simulink model "lab5machine"  (R2019b)
settings: Solver=FixedStepAuto  StartTime=0  StopTime=0.2  FixedStep=0.0001  RelTol=1e-3
values from neighbouring files (symbols this model uses):
  B = 0.01    [lab5.m]
  f = 50    [lab5.m]
  J = 0.1    [lab5.m]
  Lr = (2.2+(N/3.5e3))/1000    (= 0.00465628571429)    [lab5.m]
  Ls = (2.5+(N/4e3))/1000    (= 0.00464925)    [lab5.m]
  P = (8e3-(N/2))    (= 3701.5)    [lab5.m]
  phase = 0    [lab5.m]
  Pp = 2    [lab5.m]
  Rr = (0.3+(N/20e3))    (= 0.72985)    [lab5.m]
  Rs = (0.4+(N/15e3))    (= 0.973133333333)    [lab5.m]
  V = 400    [lab5.m]
libraries: powerlib x9
settings Model: Creator=robom  LastModifiedBy=robom
settings DataIOCC: SaveOutput=off  ReturnWorkspaceOutputs=off

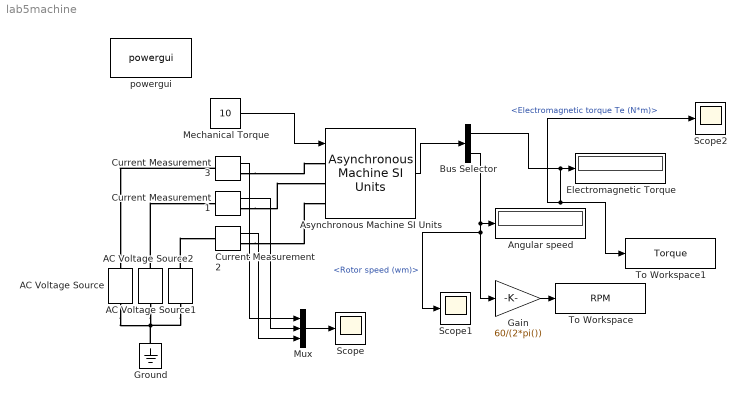
== system lab5machine ==
  AC Voltage Source : powerlib/Electrical Sources/AC Voltage Source  Amplitude=(V*sqrt(2))/sqrt(3)  Phase=phase  Frequency=f  SampleTime=0  Measurements=None  BusType=swing  Pref=10e3  Qref=0  Qmin=-inf  Qmax=+inf
      settings: SourceProductName=Simscape Electrical
  AC Voltage Source1 : powerlib/Electrical Sources/AC Voltage Source  Amplitude=(V*sqrt(2))/sqrt(3)  Phase=phase-120  Frequency=f  SampleTime=0  Measurements=None  BusType=swing  Pref=10e3  Qref=0  Qmin=-inf  Qmax=+inf
      settings: SourceProductName=Simscape Electrical
  AC Voltage Source2 : powerlib/Electrical Sources/AC Voltage Source  Amplitude=(V*sqrt(2))/sqrt(3)  Phase=phase+120  Frequency=f  SampleTime=0  Measurements=None  BusType=swing  Pref=10e3  Qref=0  Qmin=-inf  Qmax=+inf
      settings: SourceProductName=Simscape Electrical
  Angular speed : Display
  Asynchronous Machine SI Units : powerlib/Machines/Asynchronous Machine SI Units  RotorType=Squirrel-cage  PresetModel=No  MechanicalLoad=Torque Tm  ShowDetailedParameters=on  ReferenceFrame=Synchronous  Units=SI  MeasurementBus=off  NominalParameters=[P V f]  Stator=[Rs Ls]  Rotor=[Rr Lr]  Cage1=[0.4155 0.002066]  Cage2=[0.4168 0.0003495]  Lm=Lm  Mechanical=[J B Pp]  PolePairs=2  InitialConditions=[0 0 0 0 0 0 0 0]  SimulateSaturation=off  Saturation=[14.03593122, 27.81365428, 53.79336849, 72.68890987, 97.98006896, 148.6815601, 215.7428561, 302.9841135, 428.7778367 ; 230, 322, 414, 460, 506, 552, 598, 644, 690]  LoadFlowParameters=1492000  TsPowergui=0  TsBlock=-1  IterativeModel=Trapezoidal non iterative  IterativeDiscreteModel=Trapezoidal non iterative  Pmec=1.492e+006
      settings: SourceProductName=Simscape Electrical
  Bus Selector : BusSelector  OutputSignals=Mechanical.Electromagnetic torque Te (N*m),Mechanical.Rotor speed (wm)
  Current Measurement1 : powerlib/Measurements/Current Measurement  PhasorSimulation=off  OutputType=Complex  PSBequivalent=0
      settings: SourceProductName=Simscape Electrical
  Current Measurement2 : powerlib/Measurements/Current Measurement  PhasorSimulation=off  OutputType=Complex  PSBequivalent=0
      settings: SourceProductName=Simscape Electrical
  Current Measurement3 : powerlib/Measurements/Current Measurement  PhasorSimulation=off  OutputType=Complex  PSBequivalent=0
      settings: SourceProductName=Simscape Electrical
  Electromagnetic Torque : Display
  Gain : Gain  Gain=60/(2*pi())
  Ground : powerlib/Elements/Ground  LConnTagsString=a
      settings: SourceProductName=Simscape Electrical
  Mechanical Torque : Constant  Value=10
  Mux : Mux  Inputs=3
  Scope : Scope
  Scope1 : Scope
  Scope2 : Scope
  To Workspace : ToWorkspace  VariableName=RPM  SampleTime=-1
      settings: Save2DSignal=2-D array (concatenate along first dimension)
  To Workspace1 : ToWorkspace  VariableName=Torque  SampleTime=-1
      settings: Save2DSignal=2-D array (concatenate along first dimension)
  powergui : powerlib/powergui  Priority=1  SimulationMode=Continuous  SampleTime=50e-6  frequency=60  Iterations=50  frequencyindice=50  Pbase=100e6  ErrMax=1e-4  UnitsV=kV  UnitsW=MW  buscounter=0  FunctionMessages=off  echomessages=off  EnableUseOfTLC=off  CurrentSourceSwitches=off  DisableSnubberDevices=off  DisableRonSwitches=off  DisableVfSwitches=off  DisplayEquations=off  AutomaticDiscreteSolvers=off  SolverType=Tustin/Backward Euler (TBE)  Interpol=off  ExternalGateDelay=off  methode=off  Ts=100  x0status=blocks  SPID=on  SwTol=0  HookPort=off  NonlinearTolerance=1e-4  nMaxIteration=100  ContinueOnMaxIteration=off  RestoreLinks=warning  ResistiveCurrentMeasurement=off  Frange=[0:2:500]  Ylog=off  Xlog=on  ShowGrid=off  save=off  variable=ZData  structure=0  ZoomFFT=off  StartTime=0.0  cycles=1  DisplayStyle=1  fundamental=60  FreqAxis=off  MaxFrequency=1000  frequencyindicesteady=1  RmsSteady=1  display=off
      settings: SourceProductName=Simscape Electrical
  wires:
  Mechanical Torque/1 -> Asynchronous Machine SI Units/1
  Current Measurement2/1 -> Mux/3
  Current Measurement1/1 -> Mux/2
  Mux/1 -> Scope/1
  Asynchronous Machine SI Units/1 -> Bus Selector/1
  Bus Selector/1 -> To Workspace1/1, Scope2/1, Electromagnetic Torque/1  "<Electromagnetic torque Te (N*m)>"
  Bus Selector/2 -> Scope1/1, Gain/1, Angular speed/1  "<Rotor speed (wm)>"
  Current Measurement3/1 -> Mux/1
  Gain/1 -> To Workspace/1
  connections:
  Ground/LConn1 -- AC Voltage Source2/LConn1 -- AC Voltage Source1/LConn1 -- AC Voltage Source/LConn1
  AC Voltage Source2/RConn1 -- Current Measurement2/LConn1
  AC Voltage Source1/RConn1 -- Current Measurement1/LConn1
  Current Measurement3/LConn1 -- AC Voltage Source/RConn1
  Current Measurement3/RConn1 -- Asynchronous Machine SI Units/LConn1
  Current Measurement1/RConn1 -- Asynchronous Machine SI Units/LConn2
  Current Measurement2/RConn1 -- Asynchronous Machine SI Units/LConn3
